simulink model "net_mpc"  (R2018a)
settings: Solver=VariableStepAuto  StartTime=0.0  StopTime=10.0  RelTol=1e-3
libraries: neural x171
(part 4 of 7)

== system net_mpc/Cascade-Forward Neural Network/Layer 3/Delays 1 ==
  "p{3}" : Inport  PortDimensions=9
      mask Display: e = 0.06;c1 = [120 230 180]/255;c2 = ([120 230 180]+0)/(256+128);c3 = ([120 230 180]+128)/(256+128);patch([0 1 1 0],[0 0 1 1],c1);patch([0 1 1 1-e 1-e 0+e],[0 0 1 1-e 0+e 0+e],c2);patch([0 0 1 1-e 0+e 0+e],[0 1 1 1-e 1-e 0+e],c3);plot([0 1 1 0 0],[0 0 1 1 0]);
  mux : Mux  Inputs=1
      mask Display: e = 0.06;c1 = [120 150 230]/255;c2 = ([120 150 230]+0)/383;c3 = ([120 150 230]+128)/383;patch([0 1 1 0],[0 0 1 1],c1);patch([0 1 1 1-e 1-e 0+e],[0 0 1 1-e 0+e 0+e],c2);patch([0 0 1 1-e 0+e 0+e],[0 1 1 1-e 1-e 0+e],c3);plot([0 1 1 0 0],[0 0 1 1 0]);disp('Mux')
  "pd{3,1}" : Outport
      mask Display: e = 0.06;c1 = [120 230 180]/255;c2 = ([120 230 180]+0)/(256+128);c3 = ([120 230 180]+128)/(256+128);patch([0 1 1 0],[0 0 1 1],c1);patch([0 1 1 1-e 1-e 0+e],[0 0 1 1-e 0+e 0+e],c2);patch([0 0 1 1-e 0+e 0+e],[0 1 1 1-e 1-e 0+e],c3);plot([0 1 1 0 0],[0 0 1 1 0]);
  wires:
  "p{3}"/1 -> mux/1
  mux/1 -> "pd{3,1}"/1

== system net_mpc/Cascade-Forward Neural Network/Layer 3/Delays 2 ==
  "p{3}" : Inport  PortDimensions=20
      mask Display: e = 0.06;c1 = [120 230 180]/255;c2 = ([120 230 180]+0)/(256+128);c3 = ([120 230 180]+128)/(256+128);patch([0 1 1 0],[0 0 1 1],c1);patch([0 1 1 1-e 1-e 0+e],[0 0 1 1-e 0+e 0+e],c2);patch([0 0 1 1-e 0+e 0+e],[0 1 1 1-e 1-e 0+e],c3);plot([0 1 1 0 0],[0 0 1 1 0]);
  mux : Mux  Inputs=1
      mask Display: e = 0.06;c1 = [120 150 230]/255;c2 = ([120 150 230]+0)/383;c3 = ([120 150 230]+128)/383;patch([0 1 1 0],[0 0 1 1],c1);patch([0 1 1 1-e 1-e 0+e],[0 0 1 1-e 0+e 0+e],c2);patch([0 0 1 1-e 0+e 0+e],[0 1 1 1-e 1-e 0+e],c3);plot([0 1 1 0 0],[0 0 1 1 0]);disp('Mux')
  "pd{3,1}" : Outport
      mask Display: e = 0.06;c1 = [120 230 180]/255;c2 = ([120 230 180]+0)/(256+128);c3 = ([120 230 180]+128)/(256+128);patch([0 1 1 0],[0 0 1 1],c1);patch([0 1 1 1-e 1-e 0+e],[0 0 1 1-e 0+e 0+e],c2);patch([0 0 1 1-e 0+e 0+e],[0 1 1 1-e 1-e 0+e],c3);plot([0 1 1 0 0],[0 0 1 1 0]);
  wires:
  "p{3}"/1 -> mux/1
  mux/1 -> "pd{3,1}"/1

== system net_mpc/Cascade-Forward Neural Network/Layer 3/Delays 3 ==
  "p{3}" : Inport  PortDimensions=40
      mask Display: e = 0.06;c1 = [120 230 180]/255;c2 = ([120 230 180]+0)/(256+128);c3 = ([120 230 180]+128)/(256+128);patch([0 1 1 0],[0 0 1 1],c1);patch([0 1 1 1-e 1-e 0+e],[0 0 1 1-e 0+e 0+e],c2);patch([0 0 1 1-e 0+e 0+e],[0 1 1 1-e 1-e 0+e],c3);plot([0 1 1 0 0],[0 0 1 1 0]);
  mux : Mux  Inputs=1
      mask Display: e = 0.06;c1 = [120 150 230]/255;c2 = ([120 150 230]+0)/383;c3 = ([120 150 230]+128)/383;patch([0 1 1 0],[0 0 1 1],c1);patch([0 1 1 1-e 1-e 0+e],[0 0 1 1-e 0+e 0+e],c2);patch([0 0 1 1-e 0+e 0+e],[0 1 1 1-e 1-e 0+e],c3);plot([0 1 1 0 0],[0 0 1 1 0]);disp('Mux')
  "pd{3,2}" : Outport
      mask Display: e = 0.06;c1 = [120 230 180]/255;c2 = ([120 230 180]+0)/(256+128);c3 = ([120 230 180]+128)/(256+128);patch([0 1 1 0],[0 0 1 1],c1);patch([0 1 1 1-e 1-e 0+e],[0 0 1 1-e 0+e 0+e],c2);patch([0 0 1 1-e 0+e 0+e],[0 1 1 1-e 1-e 0+e],c3);plot([0 1 1 0 0],[0 0 1 1 0]);
  wires:
  "p{3}"/1 -> mux/1
  mux/1 -> "pd{3,2}"/1

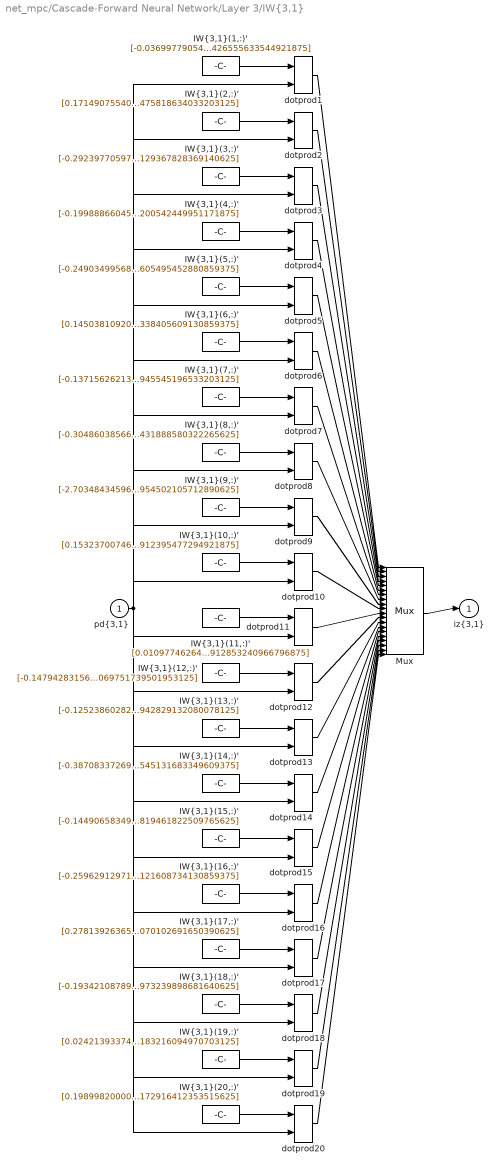
== system net_mpc/Cascade-Forward Neural Network/Layer 3/IW{3,1} ==
  "pd{3,1}" : Inport  PortDimensions=9
      mask Display: e = 0.06;c1 = [120 230 180]/255;c2 = ([120 230 180]+0)/(256+128);c3 = ([120 230 180]+128)/(256+128);patch([0 1 1 0],[0 0 1 1],c1);patch([0 1 1 1-e 1-e 0+e],[0 0 1 1-e 0+e 0+e],c2);patch([0 0 1 1-e 0+e 0+e],[0 1 1 1-e 1-e 0+e],c3);plot([0 1 1 0 0],[0 0 1 1 0]);
  "IW{3,1}(1,:)'" : Constant  Value=[-0.0369977905475218638020606931604561395943164825439453125;-0.1814618111872595973554922466064454056322574615478515625;-0.29465635189526995230124839508789591491222381591796875;-0.16720975310671148950092401719302870333194732666015625;-0.257536891246349430861783957880106754601001739501953125;0.1764165009884643697812833806892740540206432342529296875;0.2089737781923423354246693861568928696215152740478515625;0.05971184877000046409278866121894679963588714599609375;0.28045740381072625790892516306485049426555633544921875]
      mask Display: e = 0.06;c1 = [120 150 230]/255;c2 = ([120 150 230]+0)/383;c3 = ([120 150 230]+128)/383;patch([0 1 1 0],[0 0 1 1],c1);patch([0 1 1 1-e 1-e 0+e],[0 0 1 1-e 0+e 0+e],c2);patch([0 0 1 1-e 0+e 0+e],[0 1 1 1-e 1-e 0+e],c3);plot([0 1 1 0 0],[0 0 1 1 0]);disp('Weights');
  "IW{3,1}(10,:)'" : Constant  Value=[0.1532370074676365490073948194549302570521831512451171875;-0.095759157610415090999822496087290346622467041015625;0.10976140081796274816650083039348828606307506561279296875;-0.268160083274604110759042896461323834955692291259765625;-0.1131920325827235618287858187613892368972301483154296875;-0.192296831256019540301593906406196765601634979248046875;-0.2036281160807307533122667564384755678474903106689453125;-0.0305642043735486479416607608072808943688869476318359375;0.1410735802476778821823444332039798609912395477294921875]
      mask Display: e = 0.06;c1 = [120 150 230]/255;c2 = ([120 150 230]+0)/383;c3 = ([120 150 230]+128)/383;patch([0 1 1 0],[0 0 1 1],c1);patch([0 1 1 1-e 1-e 0+e],[0 0 1 1-e 0+e 0+e],c2);patch([0 0 1 1-e 0+e 0+e],[0 1 1 1-e 1-e 0+e],c3);plot([0 1 1 0 0],[0 0 1 1 0]);disp('Weights');
  "IW{3,1}(11,:)'" : Constant  Value=[0.01097746264326417316159467674197003361769020557403564453125;0.11839357647972516274226251198342652060091495513916015625;-0.361413882456698865031086143062566407024860382080078125;-0.00129825760992694524791069010660748972441069781780242919921875;0.15628538850160633710828506082179956138134002685546875;-0.2042766945934265387929684720802470110356807708740234375;0.1606225422447897788202908486709930002689361572265625;-0.293308812039141775240835841032094322144985198974609375;-0.25367750044801329334376305268961004912853240966796875]
      mask Display: e = 0.06;c1 = [120 150 230]/255;c2 = ([120 150 230]+0)/383;c3 = ([120 150 230]+128)/383;patch([0 1 1 0],[0 0 1 1],c1);patch([0 1 1 1-e 1-e 0+e],[0 0 1 1-e 0+e 0+e],c2);patch([0 0 1 1-e 0+e 0+e],[0 1 1 1-e 1-e 0+e],c3);plot([0 1 1 0 0],[0 0 1 1 0]);disp('Weights');
  "IW{3,1}(12,:)'" : Constant  Value=[-0.147942831562798027267291445241426117718219757080078125;-0.043117474060526246593116894700870034284889698028564453125;0.19462881539844867351263246746384538710117340087890625;0.09614815108351104644412998823099769651889801025390625;0.1192628328090584999277012911989004351198673248291015625;-0.3920160059707205046919398228055797517299652099609375;0.1712159511123132749066400037918356247246265411376953125;-0.130063961828653484875673029819154180586338043212890625;0.1442971862765578539011812608805485069751739501953125]
      mask Display: e = 0.06;c1 = [120 150 230]/255;c2 = ([120 150 230]+0)/383;c3 = ([120 150 230]+128)/383;patch([0 1 1 0],[0 0 1 1],c1);patch([0 1 1 1-e 1-e 0+e],[0 0 1 1-e 0+e 0+e],c2);patch([0 0 1 1-e 0+e 0+e],[0 1 1 1-e 1-e 0+e],c3);plot([0 1 1 0 0],[0 0 1 1 0]);disp('Weights');
  "IW{3,1}(13,:)'" : Constant  Value=[-0.125238602826901856968078163845348171889781951904296875;-0.06907384565921222130402412631156039424240589141845703125;-0.01443553129248955659014175267884638742543756961822509765625;-0.04308885354805284950696631085520493797957897186279296875;0.226049482345582919418092160412925295531749725341796875;-0.071301529587577128221909106287057511508464813232421875;-0.035257407282089571476380029935171478427946567535400390625;0.317958107930994493539600398435140959918498992919921875;-0.18038309778145411588212709830258972942829132080078125]
      mask Display: e = 0.06;c1 = [120 150 230]/255;c2 = ([120 150 230]+0)/383;c3 = ([120 150 230]+128)/383;patch([0 1 1 0],[0 0 1 1],c1);patch([0 1 1 1-e 1-e 0+e],[0 0 1 1-e 0+e 0+e],c2);patch([0 0 1 1-e 0+e 0+e],[0 1 1 1-e 1-e 0+e],c3);plot([0 1 1 0 0],[0 0 1 1 0]);disp('Weights');
  "IW{3,1}(14,:)'" : Constant  Value=[-0.387083372699908945246960456643137149512767791748046875;-0.326244480270388326204056284041143953800201416015625;0.08688835089162934288697925921951537020504474639892578125;-0.10966761616227020670333303087318199686706066131591796875;0.1919413346771530470835642745441873557865619659423828125;0.312026160925460482875593015705817379057407379150390625;-0.386343355232853291614247837060247547924518585205078125;0.1567904264720580143066541722873807884752750396728515625;0.1801933260943807402210126156205660663545131683349609375]
      mask Display: e = 0.06;c1 = [120 150 230]/255;c2 = ([120 150 230]+0)/383;c3 = ([120 150 230]+128)/383;patch([0 1 1 0],[0 0 1 1],c1);patch([0 1 1 1-e 1-e 0+e],[0 0 1 1-e 0+e 0+e],c2);patch([0 0 1 1-e 0+e 0+e],[0 1 1 1-e 1-e 0+e],c3);plot([0 1 1 0 0],[0 0 1 1 0]);disp('Weights');
  "IW{3,1}(15,:)'" : Constant  Value=[-0.14490658349127294446390123994206078350543975830078125;-0.274482947178163794177407908136956393718719482421875;-0.2454948341843517789495621173045947216451168060302734375;0.1880664159579661653953763789104414172470569610595703125;0.1694609471703043268586696967759053222835063934326171875;-0.24303568721583490575000041644671000540256500244140625;-0.054989497563957885628571631286831689067184925079345703125;0.2413345117036145293099025366245768964290618896484375;-0.264213965007686957253696391489938832819461822509765625]
      mask Display: e = 0.06;c1 = [120 150 230]/255;c2 = ([120 150 230]+0)/383;c3 = ([120 150 230]+128)/383;patch([0 1 1 0],[0 0 1 1],c1);patch([0 1 1 1-e 1-e 0+e],[0 0 1 1-e 0+e 0+e],c2);patch([0 0 1 1-e 0+e 0+e],[0 1 1 1-e 1-e 0+e],c3);plot([0 1 1 0 0],[0 0 1 1 0]);disp('Weights');
  "IW{3,1}(16,:)'" : Constant  Value=[-0.259629129715710338377476773530361242592334747314453125;0.1644960458853547968782748966987128369510173797607421875;0.10886698784374947146513790130484267137944698333740234375;0.044951390083088960114565679759834893047809600830078125;-0.1280213205501929130125660094563500024378299713134765625;0.160115456170731473850565862449002452194690704345703125;0.2916950837944811691926361163496039807796478271484375;0.255148878154136615759028927641338668763637542724609375;0.0243679283747323636999393414726000628434121608734130859375]
      mask Display: e = 0.06;c1 = [120 150 230]/255;c2 = ([120 150 230]+0)/383;c3 = ([120 150 230]+128)/383;patch([0 1 1 0],[0 0 1 1],c1);patch([0 1 1 1-e 1-e 0+e],[0 0 1 1-e 0+e 0+e],c2);patch([0 0 1 1-e 0+e 0+e],[0 1 1 1-e 1-e 0+e],c3);plot([0 1 1 0 0],[0 0 1 1 0]);disp('Weights');
  "IW{3,1}(17,:)'" : Constant  Value=[0.27813926365795305084560595787479542195796966552734375;0.00995378426745482068616066584354484803043305873870849609375;0.165292102812554408952649964703596197068691253662109375;0.01283456148674966268430353011353872716426849365234375;0.33206473864316754518455354627803899347782135009765625;0.30489455099222639855582883683382533490657806396484375;-0.0169136342288693890256734420063366997055709362030029296875;-0.1345267083605346247754397381868329830467700958251953125;-0.07446701484771713064336751131122582592070102691650390625]
      mask Display: e = 0.06;c1 = [120 150 230]/255;c2 = ([120 150 230]+0)/383;c3 = ([120 150 230]+128)/383;patch([0 1 1 0],[0 0 1 1],c1);patch([0 1 1 1-e 1-e 0+e],[0 0 1 1-e 0+e 0+e],c2);patch([0 0 1 1-e 0+e 0+e],[0 1 1 1-e 1-e 0+e],c3);plot([0 1 1 0 0],[0 0 1 1 0]);disp('Weights');
  "IW{3,1}(18,:)'" : Constant  Value=[-0.193421087893618615094482038330170325934886932373046875;-0.2184118530143972225499027217665570788085460662841796875;-0.213340577022640587312451998514006845653057098388671875;0.10817280965970092754258047307303058914840221405029296875;-0.08952085674493626132885992774390615522861480712890625;-0.1923411810986004055745723917425493709743022918701171875;0.1992494193953877335001578785522724501788616180419921875;-0.37687450879340966825026271180831827223300933837890625;0.043527945130068135259904238409944809973239898681640625]
      mask Display: e = 0.06;c1 = [120 150 230]/255;c2 = ([120 150 230]+0)/383;c3 = ([120 150 230]+128)/383;patch([0 1 1 0],[0 0 1 1],c1);patch([0 1 1 1-e 1-e 0+e],[0 0 1 1-e 0+e 0+e],c2);patch([0 0 1 1-e 0+e 0+e],[0 1 1 1-e 1-e 0+e],c3);plot([0 1 1 0 0],[0 0 1 1 0]);disp('Weights');
  "IW{3,1}(19,:)'" : Constant  Value=[0.024213933745713532574850290757240145467221736907958984375;0.040993231717226456811697943294348078779876232147216796875;0.391285959056181853465972153571783564984798431396484375;-0.02174331046891651852970284153343527577817440032958984375;0.3716914987907495859786877190344966948032379150390625;-0.1391929034770404971510515679256059229373931884765625;-0.2051037389346597461514676297156256623566150665283203125;0.217131993123046929117236913953092880547046661376953125;-0.0213280185590638445003452972059676540084183216094970703125]
      mask Display: e = 0.06;c1 = [120 150 230]/255;c2 = ([120 150 230]+0)/383;c3 = ([120 150 230]+128)/383;patch([0 1 1 0],[0 0 1 1],c1);patch([0 1 1 1-e 1-e 0+e],[0 0 1 1-e 0+e 0+e],c2);patch([0 0 1 1-e 0+e 0+e],[0 1 1 1-e 1-e 0+e],c3);plot([0 1 1 0 0],[0 0 1 1 0]);disp('Weights');
  "IW{3,1}(2,:)'" : Constant  Value=[0.1714907554046982973705581798640196211636066436767578125;0.033795010551617384042533132060270872898399829864501953125;0.24246755991875812430436099020880647003650665283203125;0.2484839390292789274017337675104499794542789459228515625;0.15939470771907604529360469314269721508026123046875;-0.199373036660818403476014282205142080783843994140625;-0.1589385793730268281453987810891703702509403228759765625;0.0098834058099512879513870444725398556329309940338134765625;-0.01553042200838804405560455990098489564843475818634033203125]
      mask Display: e = 0.06;c1 = [120 150 230]/255;c2 = ([120 150 230]+0)/383;c3 = ([120 150 230]+128)/383;patch([0 1 1 0],[0 0 1 1],c1);patch([0 1 1 1-e 1-e 0+e],[0 0 1 1-e 0+e 0+e],c2);patch([0 0 1 1-e 0+e 0+e],[0 1 1 1-e 1-e 0+e],c3);plot([0 1 1 0 0],[0 0 1 1 0]);disp('Weights');
  "IW{3,1}(20,:)'" : Constant  Value=[0.1989982000054886512874219306468148715794086456298828125;0.1673371229508321678114413089133449830114841461181640625;0.1120321229699567933124626506469212472438812255859375;0.239302686644814743832654357902356423437595367431640625;-0.0293267202164863745317280319113706354983150959014892578125;0.430980136264952295999108855539816431701183319091796875;-0.2180683489437880151484705493203364312648773193359375;-0.282104809477595974698260761215351521968841552734375;0.11714686392367314182738624595003784634172916412353515625]
      mask Display: e = 0.06;c1 = [120 150 230]/255;c2 = ([120 150 230]+0)/383;c3 = ([120 150 230]+128)/383;patch([0 1 1 0],[0 0 1 1],c1);patch([0 1 1 1-e 1-e 0+e],[0 0 1 1-e 0+e 0+e],c2);patch([0 0 1 1-e 0+e 0+e],[0 1 1 1-e 1-e 0+e],c3);plot([0 1 1 0 0],[0 0 1 1 0]);disp('Weights');
  "IW{3,1}(3,:)'" : Constant  Value=[-0.292397705977859023729337195618427358567714691162109375;-0.1163007737663808993655578660764149390161037445068359375;0.34342578300257020629260296118445694446563720703125;0.0161686766078314829442330591291465680114924907684326171875;-0.3516231515338208435395017659175209701061248779296875;-0.039530784729812397382264776979354792274534702301025390625;0.1797609147092182613203448227068292908370494842529296875;0.289031429591097233089413975903880782425403594970703125;0.160388778220906191851469202447333373129367828369140625]
      mask Display: e = 0.06;c1 = [120 150 230]/255;c2 = ([120 150 230]+0)/383;c3 = ([120 150 230]+128)/383;patch([0 1 1 0],[0 0 1 1],c1);patch([0 1 1 1-e 1-e 0+e],[0 0 1 1-e 0+e 0+e],c2);patch([0 0 1 1-e 0+e 0+e],[0 1 1 1-e 1-e 0+e],c3);plot([0 1 1 0 0],[0 0 1 1 0]);disp('Weights');
  "IW{3,1}(4,:)'" : Constant  Value=[-0.19988866045805064874940626395982690155506134033203125;0.232111023987214781794108375834184698760509490966796875;-0.0161225272437239101896988557882650638930499553680419921875;-0.1321782948279755787179823300903080962598323822021484375;0.181430842283985482854546944508911110460758209228515625;-0.1851062536420469417652867605283972807228565216064453125;-0.10851290177640653122903557914469274692237377166748046875;-0.1787843662167559466436017601154162548482418060302734375;0.1039985194372321231082167969361762516200542449951171875]
      mask Display: e = 0.06;c1 = [120 150 230]/255;c2 = ([120 150 230]+0)/383;c3 = ([120 150 230]+128)/383;patch([0 1 1 0],[0 0 1 1],c1);patch([0 1 1 1-e 1-e 0+e],[0 0 1 1-e 0+e 0+e],c2);patch([0 0 1 1-e 0+e 0+e],[0 1 1 1-e 1-e 0+e],c3);plot([0 1 1 0 0],[0 0 1 1 0]);disp('Weights');
  "IW{3,1}(5,:)'" : Constant  Value=[-0.249034995685935955922474249746301211416721343994140625;0.264406852070697973022816995580797083675861358642578125;-0.310593801346571718458022814957075752317905426025390625;-0.03868431234515150307640141136289457790553569793701171875;-0.15815880140814309040564467068179510533809661865234375;-0.21329218345218647900907171788276173174381256103515625;-0.11554320046410139488646251493264571763575077056884765625;-0.00175268098649540571276617129115038551390171051025390625;-0.0701190633999784207475158837041817605495452880859375]
      mask Display: e = 0.06;c1 = [120 150 230]/255;c2 = ([120 150 230]+0)/383;c3 = ([120 150 230]+128)/383;patch([0 1 1 0],[0 0 1 1],c1);patch([0 1 1 1-e 1-e 0+e],[0 0 1 1-e 0+e 0+e],c2);patch([0 0 1 1-e 0+e 0+e],[0 1 1 1-e 1-e 0+e],c3);plot([0 1 1 0 0],[0 0 1 1 0]);disp('Weights');
  "IW{3,1}(6,:)'" : Constant  Value=[0.1450381092015907980030675616944790817797183990478515625;-0.18098929124635443344004670507274568080902099609375;0.1651169178654978419995558169830474071204662322998046875;-0.141511365372540443008375632416573353111743927001953125;-0.0106592166803264609686863195747719146311283111572265625;-0.10866619567182254912918182299108593724668025970458984375;0.0828678979260208115054098243490443564951419830322265625;0.031799237991739968955950956797096296213567256927490234375;0.147000856967280879583626074236235581338405609130859375]
      mask Display: e = 0.06;c1 = [120 150 230]/255;c2 = ([120 150 230]+0)/383;c3 = ([120 150 230]+128)/383;patch([0 1 1 0],[0 0 1 1],c1);patch([0 1 1 1-e 1-e 0+e],[0 0 1 1-e 0+e 0+e],c2);patch([0 0 1 1-e 0+e 0+e],[0 1 1 1-e 1-e 0+e],c3);plot([0 1 1 0 0],[0 0 1 1 0]);disp('Weights');
  "IW{3,1}(7,:)'" : Constant  Value=[-0.13715626213002707345367525704205036163330078125;-0.077912876643881523452961346265510655939579010009765625;-0.07578870389226277648475615933421067893505096435546875;0.2581260341174969052957521853386424481868743896484375;0.22058844448637426882697809560340829193592071533203125;0.057721963613241056290092956260195933282375335693359375;0.0707038640896352765796706307810381986200809478759765625;-0.2264505701653647395943380615790374577045440673828125;0.101737818028696136440913733167690224945545196533203125]
      mask Display: e = 0.06;c1 = [120 150 230]/255;c2 = ([120 150 230]+0)/383;c3 = ([120 150 230]+128)/383;patch([0 1 1 0],[0 0 1 1],c1);patch([0 1 1 1-e 1-e 0+e],[0 0 1 1-e 0+e 0+e],c2);patch([0 0 1 1-e 0+e 0+e],[0 1 1 1-e 1-e 0+e],c3);plot([0 1 1 0 0],[0 0 1 1 0]);disp('Weights');
  "IW{3,1}(8,:)'" : Constant  Value=[-0.304860385664164901253769812683458440005779266357421875;0.178057058389677502763248639894300140440464019775390625;0.2090419849934667950730471375209162943065166473388671875;0.0360992652837159588852244951340253464877605438232421875;-0.29566465112279727289745778762153349816799163818359375;0.256212430120864975702232868570717982947826385498046875;0.13862101079022626226588954523322172462940216064453125;0.1311068225323110680857752186057041399180889129638671875;-0.212664380117378704060371319428668357431888580322265625]
      mask Display: e = 0.06;c1 = [120 150 230]/255;c2 = ([120 150 230]+0)/383;c3 = ([120 150 230]+128)/383;patch([0 1 1 0],[0 0 1 1],c1);patch([0 1 1 1-e 1-e 0+e],[0 0 1 1-e 0+e 0+e],c2);patch([0 0 1 1-e 0+e 0+e],[0 1 1 1-e 1-e 0+e],c3);plot([0 1 1 0 0],[0 0 1 1 0]);disp('Weights');
  "IW{3,1}(9,:)'" : Constant  Value=[-2.703484345969691510745691598316398085444234311580657958984375e-05;-0.17100255176231071718717657859087921679019927978515625;0.03348720886013044351070533366510062478482723236083984375;0.353803228175260386922929001229931600391864776611328125;0.191421632692522047936023454894893802702426910400390625;-0.162584856375183328669464799531851895153522491455078125;-0.32817058942934640430877379912999458611011505126953125;0.269198845364432115534469858175725676119327545166015625;-0.1780056950084471234507788039991282857954502105712890625]
      mask Display: e = 0.06;c1 = [120 150 230]/255;c2 = ([120 150 230]+0)/383;c3 = ([120 150 230]+128)/383;patch([0 1 1 0],[0 0 1 1],c1);patch([0 1 1 1-e 1-e 0+e],[0 0 1 1-e 0+e 0+e],c2);patch([0 0 1 1-e 0+e 0+e],[0 1 1 1-e 1-e 0+e],c3);plot([0 1 1 0 0],[0 0 1 1 0]);disp('Weights');
  Mux : Mux  Inputs=20
      mask Display: e = 0.06;c1 = [120 150 230]/255;c2 = ([120 150 230]+0)/383;c3 = ([120 150 230]+128)/383;patch([0 1 1 0],[0 0 1 1],c1);patch([0 1 1 1-e 1-e 0+e],[0 0 1 1-e 0+e 0+e],c2);patch([0 0 1 1-e 0+e 0+e],[0 1 1 1-e 1-e 0+e],c3);plot([0 1 1 0 0],[0 0 1 1 0]);disp('Mux');
  dotprod{1..20} (20 alike) : neural/Weight Functions/dotprod
  "iz{3,1}" : Outport
      mask Display: e = 0.06;c1 = [120 230 180]/255;c2 = ([120 230 180]+0)/(256+128);c3 = ([120 230 180]+128)/(256+128);patch([0 1 1 0],[0 0 1 1],c1);patch([0 1 1 1-e 1-e 0+e],[0 0 1 1-e 0+e 0+e],c2);patch([0 0 1 1-e 0+e 0+e],[0 1 1 1-e 1-e 0+e],c3);plot([0 1 1 0 0],[0 0 1 1 0]);
  wires:
  "IW{3,1}(1,:)'"/1 -> dotprod1/1
  "pd{3,1}"/1 -> dotprod1/2, dotprod2/2, dotprod3/2, dotprod4/2, dotprod5/2, dotprod6/2, dotprod7/2, dotprod8/2, dotprod9/2, dotprod10/2, dotprod11/2, dotprod12/2, dotprod13/2, dotprod14/2, dotprod15/2, dotprod16/2, dotprod17/2, dotprod18/2, dotprod19/2, dotprod20/2
  dotprod1/1 -> Mux/1
  "IW{3,1}(2,:)'"/1 -> dotprod2/1
  dotprod2/1 -> Mux/2
  "IW{3,1}(3,:)'"/1 -> dotprod3/1
  dotprod3/1 -> Mux/3
  "IW{3,1}(4,:)'"/1 -> dotprod4/1
  dotprod4/1 -> Mux/4
  "IW{3,1}(5,:)'"/1 -> dotprod5/1
  dotprod5/1 -> Mux/5
  "IW{3,1}(6,:)'"/1 -> dotprod6/1
  dotprod6/1 -> Mux/6
  "IW{3,1}(7,:)'"/1 -> dotprod7/1
  dotprod7/1 -> Mux/7
  "IW{3,1}(8,:)'"/1 -> dotprod8/1
  dotprod8/1 -> Mux/8
  "IW{3,1}(9,:)'"/1 -> dotprod9/1
  dotprod9/1 -> Mux/9
  "IW{3,1}(10,:)'"/1 -> dotprod10/1
  dotprod10/1 -> Mux/10
  "IW{3,1}(11,:)'"/1 -> dotprod11/1
  dotprod11/1 -> Mux/11
  "IW{3,1}(12,:)'"/1 -> dotprod12/1
  dotprod12/1 -> Mux/12
  "IW{3,1}(13,:)'"/1 -> dotprod13/1
  dotprod13/1 -> Mux/13
  "IW{3,1}(14,:)'"/1 -> dotprod14/1
  dotprod14/1 -> Mux/14
  "IW{3,1}(15,:)'"/1 -> dotprod15/1
  dotprod15/1 -> Mux/15
  "IW{3,1}(16,:)'"/1 -> dotprod16/1
  dotprod16/1 -> Mux/16
  "IW{3,1}(17,:)'"/1 -> dotprod17/1
  dotprod17/1 -> Mux/17
  "IW{3,1}(18,:)'"/1 -> dotprod18/1
  dotprod18/1 -> Mux/18
  "IW{3,1}(19,:)'"/1 -> dotprod19/1
  dotprod19/1 -> Mux/19
  "IW{3,1}(20,:)'"/1 -> dotprod20/1
  dotprod20/1 -> Mux/20
  Mux/1 -> "iz{3,1}"/1
